simulink model "sampleModel2072_pp_difftest"  (R2021a)
settings: Solver=VariableStepAuto  StartTime=0.0  StopTime=10.0  RelTol=1e-3
undefined symbols (not defined in the file or in its folder): DiscIntNeverNeededParam, magnitude, Newton, Raphson
libraries: simulink x184, pid_lib x33
(part 4 of 5)

== system sampleModel2072_pp_difftest/cfblk49/cfblk12 ==
  cfblk1 : Inport
  cfblk3 : pid_lib/PID Controller  Controller=PID  Form=Parallel  TimeDomain=Discrete-time  UseExternalTs=off  SampleTime=1  IntegratorMethod=Forward Euler  FilterMethod=Forward Euler  ControllerParametersSource=internal  P=1  I=1  D=0  UseFilter=on  N=100  TunerSelectOption=Transfer Function Based (PID Tuner App)  InitialConditionSource=internal  InitialConditionForIntegrator=0  InitialConditionForFilter=0  DifferentiatorICPrevScaledInput=0  ExternalReset=none  TrackingMode=off  Kt=1  LimitOutput=off  SatLimitsSource=internal  UpperSaturationLimit=inf  LowerSaturationLimit=-inf  LinearizeAsGain=off  AntiWindupMode=none  Kb=1  POutMin=[]  POutMax=[]  IOutMin=[]  IOutMax=[]  DOutMin=[]  DOutMax=[]  NOutMin=[]  NOutMax=[]  SumOutMin=[]  SumOutMax=[]  SaturationOutMin=[]  SaturationOutMax=[]  PParamMin=[]  PParamMax=[]  IParamMin=[]  IParamMax=[]  DParamMin=[]  DParamMax=[]  NParamMin=[]  NParamMax=[]  KbParamMin=[]  KbParamMax=[]  KtParamMin=[]  KtParamMax=[]  KbOutMin=[]  KbOutMax=[]  KtOutMin=[]  KtOutMax=[]  IntegratorOutMin=[]  IntegratorOutMax=[]  FilterOutMin=[]  FilterOutMax=[]  SumI1OutMin=[]  SumI1OutMax=[]  SumI2OutMin=[]  SumI2OutMax=[]  SumI3OutMin=[]  SumI3OutMax=[]  SumI4OutMin=[]  SumI4OutMax=[]  SumDOutMin=[]  SumDOutMax=[]  DifferentiatorOutMin=[]  DifferentiatorOutMax=[]  FilterDiffOutCoefMin=[]  FilterDiffOutCoefMax=[]  ReciprocalOutMin=[]  ReciprocalOutMax=[]  SumDenOutMin=[]  SumDenOutMax=[]  SumNumOutMin=[]  SumNumOutMax=[]  DivideOutMin=[]  DivideOutMax=[]  UdiffTsProdOutMin=[]  UdiffTsProdOutMax=[]  NTsProdOutMin=[]  NTsProdOutMax=[]  UintegralTsProdOutMin=[]  UintegralTsProdOutMax=[]  UngainTsProdOutMin=[]  UngainTsProdOutMax=[]  IntegratorContinuousStateAttributes=''  IntegratorStateMustResolveToSignalObject=off  IntegratorRTWStateStorageClass=Auto  FilterContinuousStateAttributes=''  FilterStateMustResolveToSignalObject=off  FilterRTWStateStorageClass=Auto  ParallelPVariant=InternalParameters  IdealPVariant=Disabled  IVariant=InternalParameters  DVariant=InternalParameters  IntegratorVariant=Discrete  SatVariant=Disabled  AWVariant=Passthrough  PCopyVariant=Disabled  TRVariant=Disabled  FdbkBlocksVariant=Forward  IdealPFdbkVariant=Disabled  SatFdbkVariant=Disabled  DerivativeFilterVariant=ForwardEulerFilter  NVariant=InternalParameters  NCopyVariant=Disabled  FilterICVariant=InternalICsFilter  IntegratorICVariant=InternalICs  ExternalResetVariant=Disabled  TRSumVariant=Passthrough  SumFdbkVariant=Disabled  SumVariant=Sum_PID  TsampFilterVariant=InternalTs  TsampNgainVariant=Passthrough  TsampIntegralVariant=Passthrough  ExternalSaturationOutDataTypeStr=Inherit: Same as second input
  cfblk4 : simulink/Discrete/Transfer Fcn Lead or Lag  PoleZ=0.95  ZeroZ=0.75  ICPrevOutput=0.0  ICPrevInput=0.0  DoSatur=off
      settings: SourceProductBaseCode=SL
  cfblk5 : Abs
  cfblk6 : Math  Operator=mod  SaturateOnIntegerOverflow=on
  cfblk7 : Squeeze
  cfblk8 : Delay  SampleTime=1
  cfblk2 : Outport
  wires:
  cfblk6/1 -> cfblk3/1
  cfblk5/1 -> cfblk2/1
  cfblk3/1 -> cfblk7/1
  cfblk7/1 -> cfblk4/1, cfblk5/1
  cfblk1/1 -> cfblk6/2
  cfblk4/1 -> cfblk8/1
  cfblk8/1 -> cfblk6/1

== system sampleModel2072_pp_difftest/cfblk49/cfblk13 ==
  cfblk1 : Inport
  cfblk3 : DiscreteTransferFcn  SampleTime=1
  cfblk4 : simulink/Discrete/Difference  ICPrevInput=0.0  OutMin=[]  OutMax=[]  OutDataTypeStr=Inherit: Inherit via back propagation  OutDataType=fixdt(1, 16)  OutScaling=2^-10  DoSatur=off
  cfblk5 : Polyval  Coefs=[ +2.081618890e-019, -1.441693666e-014, +4.719686976e-010, -8.536869453e-006, +1.621573104e-001, -8.087801117e+001 ]
  cfblk6 : Product  Inputs=**
  cfblk7 : MinMax
  cfblk8 : Sin  TimeSource=Use external signal  SampleTime=0
  cfblk9 : Constant  Value=[-889653633.727904]  SampleTime=1
  cfblk2 : Outport
  wires:
  cfblk1/1 -> cfblk6/1
  cfblk9/1 -> cfblk3/1
  cfblk7/1 -> cfblk6/2
  cfblk6/1 -> cfblk2/1
  cfblk8/1 -> cfblk7/1
  cfblk3/1 -> cfblk5/1, cfblk4/1
  cfblk5/1 -> cfblk8/1

== system sampleModel2072_pp_difftest/cfblk49/cfblk14 ==
  cfblk1 : Inport
  cfblk10 : ComplexToRealImag
  cfblk11 : Polyval  Coefs=[ +2.081618890e-019, -1.441693666e-014, +4.719686976e-010, -8.536869453e-006, +1.621573104e-001, -8.087801117e+001 ]
  cfblk12 : Product
  cfblk13 : Reshape
  cfblk14 : Delay  SampleTime=1
  cfblk15 : Delay  SampleTime=1
  cfblk3 : DiscreteStateSpace
  cfblk4 : pid_lib/PID Controller (2DOF)  Controller=PID  Form=Parallel  TimeDomain=Discrete-time  UseExternalTs=off  SampleTime=1  IntegratorMethod=Forward Euler  FilterMethod=Forward Euler  ControllerParametersSource=internal  P=1  I=1  D=0  UseFilter=on  N=100  b=1  c=1  TunerSelectOption=Transfer Function Based (PID Tuner App)  InitialConditionSource=internal  InitialConditionForIntegrator=0  InitialConditionForFilter=0  DifferentiatorICPrevScaledInput=0  ExternalReset=none  TrackingMode=off  Kt=1  LimitOutput=off  SatLimitsSource=internal  UpperSaturationLimit=inf  LowerSaturationLimit=-inf  LinearizeAsGain=off  AntiWindupMode=none  Kb=1  POutMin=[]  POutMax=[]  IOutMin=[]  IOutMax=[]  DOutMin=[]  DOutMax=[]  NOutMin=[]  NOutMax=[]  bOutMin=[]  bOutMax=[]  cOutMin=[]  cOutMax=[]  SumOutMin=[]  SumOutMax=[]  SaturationOutMin=[]  SaturationOutMax=[]  PParamMin=[]  PParamMax=[]  IParamMin=[]  IParamMax=[]  DParamMin=[]  DParamMax=[]  NParamMin=[]  NParamMax=[]  bParamMin=[]  bParamMax=[]  cParamMin=[]  cParamMax=[]  KbParamMin=[]  KbParamMax=[]  KtParamMin=[]  KtParamMax=[]  KbOutMin=[]  KbOutMax=[]  KtOutMin=[]  KtOutMax=[]  IntegratorOutMin=[]  IntegratorOutMax=[]  FilterOutMin=[]  FilterOutMax=[]  SumI1OutMin=[]  SumI1OutMax=[]  SumI2OutMin=[]  SumI2OutMax=[]  SumI3OutMin=[]  SumI3OutMax=[]  SumI4OutMin=[]  SumI4OutMax=[]  SumDOutMin=[]  SumDOutMax=[]  Sum1OutMin=[]  Sum1OutMax=[]  Sum2OutMin=[]  Sum2OutMax=[]  Sum3OutMin=[]  Sum3OutMax=[]  DifferentiatorOutMin=[]  DifferentiatorOutMax=[]  FilterDiffOutCoefMin=[]  FilterDiffOutCoefMax=[]  ReciprocalOutMin=[]  ReciprocalOutMax=[]  SumDenOutMin=[]  SumDenOutMax=[]  SumNumOutMin=[]  SumNumOutMax=[]  DivideOutMin=[]  DivideOutMax=[]  UdiffTsProdOutMin=[]  UdiffTsProdOutMax=[]  NTsProdOutMin=[]  NTsProdOutMax=[]  UintegralTsProdOutMin=[]  UintegralTsProdOutMax=[]  UngainTsProdOutMin=[]  UngainTsProdOutMax=[]  IntegratorContinuousStateAttributes=''  IntegratorStateMustResolveToSignalObject=off  IntegratorRTWStateStorageClass=Auto  FilterContinuousStateAttributes=''  FilterStateMustResolveToSignalObject=off  FilterRTWStateStorageClass=Auto  ParallelPVariant=InternalParameters  IdealPVariant=Disabled  IVariant=InternalParameters  DVariant=InternalParameters  bVariant=InternalParameters  cVariant=InternalParameters  IntegratorVariant=Discrete  SatVariant=Disabled  AWVariant=Passthrough  PCopyVariant=Disabled  TRVariant=Disabled  FdbkBlocksVariant=Forward  IdealPFdbkVariant=Disabled  SatFdbkVariant=Disabled  DerivativeFilterVariant=ForwardEulerFilter  NVariant=InternalParameters  NCopyVariant=Disabled  FilterICVariant=InternalICsFilter  IntegratorICVariant=InternalICs  ExternalResetVariant=Disabled  TRSumVariant=Passthrough  SumFdbkVariant=Disabled  SumVariant=Sum_PID  TsampFilterVariant=InternalTs  TsampNgainVariant=Passthrough  TsampIntegralVariant=Passthrough  ExternalSaturationOutDataTypeStr=Inherit: Same as second input
      settings: SourceProductBaseCode=SL
  cfblk5 : simulink/Discrete/Transfer Fcn Real Zero  ZeroZ=0.75  ICPrevInput=0.0  DoSatur=off
      settings: SourceProductBaseCode=SL
  cfblk6 : Gain  Gain=[-781160074.490628]
  cfblk7 : Rounding
  cfblk8 : Abs
  cfblk9 : Sin  TimeSource=Use external signal  SampleTime=0
  cfblk2 : Outport
  wires:
  cfblk8/1 -> cfblk10/1
  cfblk5/1 -> cfblk13/1
  cfblk9/1 -> cfblk8/1
  cfblk4/1 -> cfblk2/1
  cfblk13/1 -> cfblk3/1, cfblk9/1
  cfblk6/1 -> cfblk4/1
  cfblk1/1 -> cfblk6/1
  cfblk11/1 -> cfblk7/1
  cfblk3/1 -> cfblk12/1
  cfblk12/1 -> cfblk11/1
  cfblk10/2 -> cfblk4/2
  cfblk7/1 -> cfblk14/1
  cfblk14/1 -> cfblk12/2
  cfblk10/1 -> cfblk15/1
  cfblk15/1 -> cfblk5/1

== system sampleModel2072_pp_difftest/cfblk49/cfblk15 ==
  cfblk1 : Inport
  cfblk11 : Inport  Port=2
  cfblk10 : Signum
  cfblk3 : UnitDelay  HasFrameUpgradeWarning=on
  cfblk4 : DiscreteFir  SampleTime=1
  cfblk5 : DiscreteZeroPole  Poles=[0 0.5]  Gain=1
  cfblk6 : Squeeze
  cfblk7 : Sqrt  SaturateOnIntegerOverflow=on
  cfblk8 : Squeeze
  cfblk9 : UnaryMinus
  cfblk2 : Outport
  wires:
  cfblk10/1 -> cfblk4/1
  cfblk3/1 -> cfblk2/1
  cfblk1/1 -> cfblk7/1
  cfblk8/1 -> cfblk5/1
  cfblk11/1 -> cfblk10/1
  cfblk5/1 -> cfblk9/1
  cfblk6/1 -> cfblk8/1
  cfblk7/1 -> cfblk6/1
  cfblk9/1 -> cfblk3/1

== system sampleModel2072_pp_difftest/cfblk49/cfblk16 ==
  cfblk1 : Inport
  cfblk10 : PermuteDimensions
  cfblk11 : Sum  Inputs=+
  cfblk12 : UnaryMinus
  cfblk13 : Sum  Inputs=+-
  cfblk14 : simulink/Math Operations/MinMax Running Resettable  Function=min  vinit=0.0
  cfblk15 : Reshape
  cfblk16 : Gain  Gain=[569641442.410553]
  cfblk17 : Delay  SampleTime=1
  cfblk18 : Delay  SampleTime=1
  cfblk3 : pid_lib/PID Controller (2DOF)  Controller=PID  Form=Parallel  TimeDomain=Discrete-time  UseExternalTs=off  SampleTime=1  IntegratorMethod=Forward Euler  FilterMethod=Forward Euler  ControllerParametersSource=internal  P=1  I=1  D=0  UseFilter=on  N=100  b=1  c=1  TunerSelectOption=Transfer Function Based (PID Tuner App)  InitialConditionSource=internal  InitialConditionForIntegrator=0  InitialConditionForFilter=0  DifferentiatorICPrevScaledInput=0  ExternalReset=none  TrackingMode=off  Kt=1  LimitOutput=off  SatLimitsSource=internal  UpperSaturationLimit=inf  LowerSaturationLimit=-inf  LinearizeAsGain=off  AntiWindupMode=none  Kb=1  POutMin=[]  POutMax=[]  IOutMin=[]  IOutMax=[]  DOutMin=[]  DOutMax=[]  NOutMin=[]  NOutMax=[]  bOutMin=[]  bOutMax=[]  cOutMin=[]  cOutMax=[]  SumOutMin=[]  SumOutMax=[]  SaturationOutMin=[]  SaturationOutMax=[]  PParamMin=[]  PParamMax=[]  IParamMin=[]  IParamMax=[]  DParamMin=[]  DParamMax=[]  NParamMin=[]  NParamMax=[]  bParamMin=[]  bParamMax=[]  cParamMin=[]  cParamMax=[]  KbParamMin=[]  KbParamMax=[]  KtParamMin=[]  KtParamMax=[]  KbOutMin=[]  KbOutMax=[]  KtOutMin=[]  KtOutMax=[]  IntegratorOutMin=[]  IntegratorOutMax=[]  FilterOutMin=[]  FilterOutMax=[]  SumI1OutMin=[]  SumI1OutMax=[]  SumI2OutMin=[]  SumI2OutMax=[]  SumI3OutMin=[]  SumI3OutMax=[]  SumI4OutMin=[]  SumI4OutMax=[]  SumDOutMin=[]  SumDOutMax=[]  Sum1OutMin=[]  Sum1OutMax=[]  Sum2OutMin=[]  Sum2OutMax=[]  Sum3OutMin=[]  Sum3OutMax=[]  DifferentiatorOutMin=[]  DifferentiatorOutMax=[]  FilterDiffOutCoefMin=[]  FilterDiffOutCoefMax=[]  ReciprocalOutMin=[]  ReciprocalOutMax=[]  SumDenOutMin=[]  SumDenOutMax=[]  SumNumOutMin=[]  SumNumOutMax=[]  DivideOutMin=[]  DivideOutMax=[]  UdiffTsProdOutMin=[]  UdiffTsProdOutMax=[]  NTsProdOutMin=[]  NTsProdOutMax=[]  UintegralTsProdOutMin=[]  UintegralTsProdOutMax=[]  UngainTsProdOutMin=[]  UngainTsProdOutMax=[]  IntegratorContinuousStateAttributes=''  IntegratorStateMustResolveToSignalObject=off  IntegratorRTWStateStorageClass=Auto  FilterContinuousStateAttributes=''  FilterStateMustResolveToSignalObject=off  FilterRTWStateStorageClass=Auto  ParallelPVariant=InternalParameters  IdealPVariant=Disabled  IVariant=InternalParameters  DVariant=InternalParameters  bVariant=InternalParameters  cVariant=InternalParameters  IntegratorVariant=Discrete  SatVariant=Disabled  AWVariant=Passthrough  PCopyVariant=Disabled  TRVariant=Disabled  FdbkBlocksVariant=Forward  IdealPFdbkVariant=Disabled  SatFdbkVariant=Disabled  DerivativeFilterVariant=ForwardEulerFilter  NVariant=InternalParameters  NCopyVariant=Disabled  FilterICVariant=InternalICsFilter  IntegratorICVariant=InternalICs  ExternalResetVariant=Disabled  TRSumVariant=Passthrough  SumFdbkVariant=Disabled  SumVariant=Sum_PID  TsampFilterVariant=InternalTs  TsampNgainVariant=Passthrough  TsampIntegralVariant=Passthrough  ExternalSaturationOutDataTypeStr=Inherit: Same as second input
      settings: SourceProductBaseCode=SL
  cfblk4 : Delay  ShowEnablePort=on  SampleTime=1
      settings: InputPortMap=u0,e6
  cfblk5 : DiscreteIntegrator  ICPrevOutput=DiscIntNeverNeededParam  ICPrevScaledInput=DiscIntNeverNeededParam
  cfblk6 : UnitDelay  HasFrameUpgradeWarning=on
  cfblk7 : Delay  ShowEnablePort=on  SampleTime=1
      settings: InputPortMap=u0,e6
  cfblk8 : Reshape
  cfblk9 : simulink/Math Operations/Slider Gain  gain=1  low=0  high=2
  cfblk2 : Outport
  wires:
  cfblk4/1 -> cfblk5/1
  cfblk14/1 -> cfblk3/1
  cfblk1/1 -> cfblk16/1, cfblk14/2
  cfblk9/1 -> cfblk11/1, cfblk8/1
  cfblk5/1 -> cfblk12/1
  cfblk8/1 -> cfblk7/1, cfblk7/2
  cfblk12/1 -> cfblk6/1
  cfblk16/1 -> cfblk3/2
  cfblk11/1 -> cfblk4/1, cfblk15/1
  cfblk13/1 -> cfblk2/1
  cfblk10/1 -> cfblk13/1
  cfblk7/1 -> cfblk14/1
  cfblk3/1 -> cfblk10/1
  cfblk6/1 -> cfblk13/2, cfblk17/1
  cfblk17/1 -> cfblk4/2
  cfblk15/1 -> cfblk18/1
  cfblk18/1 -> cfblk9/1

== system sampleModel2072_pp_difftest/cfblk49/cfblk18 ==
  cfblk1 : Inport
  cfblk15 : Inport  Port=2
  Action Port : ActionPort  ActionPortLabel=if(u1 >= 0)
  cfblk10 : UnaryMinus
  cfblk11 : Signum
  cfblk12 : Bias  Bias=[-787448639.823052]
  cfblk13 : DotProduct  InputSameDT=on  OutDataTypeStr=Inherit: Inherit via internal rule
  cfblk14 : Constant  Value=[137570796.865907]  SampleTime=1
  cfblk16 : Delay
  cfblk17 : Delay
  cfblk3 : simulink/Discrete/Tapped Delay  vinit=0.0  samptime=-1  NumDelays=1  DelayOrder=Oldest  includeCurrent=off
  cfblk4 : DiscreteFir
  cfblk5 : simulink/Discrete/Transfer Fcn Lead or Lag  PoleZ=0.95  ZeroZ=0.75  ICPrevOutput=0.0  ICPrevInput=0.0  DoSatur=off
      settings: SourceProductBaseCode=SL
  cfblk6 : Product  Inputs=**
  cfblk7 : Polyval  Coefs=[ +2.081618890e-019, -1.441693666e-014, +4.719686976e-010, -8.536869453e-006, +1.621573104e-001, -8.087801117e+001 ]
  cfblk8 : simulink/Math Operations/MinMax Running Resettable  Function=min  vinit=0.0
  cfblk9 : Squeeze
  cfblk2 : Outport
  wires:
  cfblk8/1 -> cfblk3/1
  cfblk13/1 -> cfblk7/1
  cfblk6/1 -> cfblk4/1
  cfblk10/1 -> cfblk2/1, cfblk16/1
  cfblk7/1 -> cfblk12/1
  cfblk4/1 -> cfblk10/1
  cfblk1/1 -> cfblk6/1
  cfblk15/1 -> cfblk11/1
  cfblk3/1 -> cfblk5/1
  cfblk5/1 -> cfblk9/1
  cfblk9/1 -> cfblk13/1
  cfblk11/1 -> cfblk8/1
  cfblk14/1 -> cfblk8/2
  cfblk16/1 -> cfblk6/2
  cfblk12/1 -> cfblk17/1
  cfblk17/1 -> cfblk13/2

== system sampleModel2072_pp_difftest/cfblk49/cfblk19 ==
  cfblk1 : Inport
  Action Port : ActionPort  ActionPortLabel=else
  cfblk10 : Sqrt  SaturateOnIntegerOverflow=on
  cfblk11 : Polyval  Coefs=[ +2.081618890e-019, -1.441693666e-014, +4.719686976e-010, -8.536869453e-006, +1.621573104e-001, -8.087801117e+001 ]
  cfblk12 : Product
  cfblk13 : Abs
  cfblk14 : Delay
  cfblk15 : Delay
  cfblk3 : DiscreteZeroPole  Poles=[0 0.5]  Gain=1  SampleTime=-1
  cfblk4 : Delay
  cfblk5 : DiscreteStateSpace  SampleTime=-1
  cfblk6 : Sum  Inputs=+-
  cfblk7 : Sqrt  Operator=rSqrt  AlgorithmType=Newton-Raphson  SaturateOnIntegerOverflow=on
  cfblk8 : Polyval  Coefs=[ +2.081618890e-019, -1.441693666e-014, +4.719686976e-010, -8.536869453e-006, +1.621573104e-001, -8.087801117e+001 ]
  cfblk9 : Sum  Inputs=+
  cfblk2 : Outport
  wires:
  cfblk5/1 -> cfblk9/1, cfblk4/1
  cfblk13/1 -> cfblk11/1
  cfblk12/1 -> cfblk13/1
  cfblk1/1 -> cfblk7/1
  cfblk8/1 -> cfblk2/1
  cfblk4/1 -> cfblk8/1
  cfblk7/1 -> cfblk10/1
  cfblk10/1 -> cfblk6/1, cfblk6/2
  cfblk6/1 -> cfblk12/2
  cfblk11/1 -> cfblk3/1
  cfblk3/1 -> cfblk14/1
  cfblk14/1 -> cfblk12/1
  cfblk9/1 -> cfblk15/1
  cfblk15/1 -> cfblk5/1

== system sampleModel2072_pp_difftest/cfblk51/cfblk6 ==
  cfblk1 : Inport
  cfblk10 : Sqrt  SaturateOnIntegerOverflow=on
  cfblk11 : Sqrt  SaturateOnIntegerOverflow=on
  cfblk12 : Assignment  DiagnosticForDimensions=Warning  IndexOptions=Index vector (dialog)  Indices=1  OutputSizes=1
  cfblk13 : Sqrt  SaturateOnIntegerOverflow=on
  cfblk14 : Product  Inputs=*
  cfblk15 : Delay  SampleTime=1
  cfblk16 : Delay  SampleTime=1
  cfblk17 : Delay  SampleTime=1
  cfblk3 : DiscreteStateSpace
  cfblk4 : DiscreteFir  SampleTime=1
  cfblk5 : pid_lib/PID Controller (2DOF)  Controller=PID  Form=Parallel  TimeDomain=Discrete-time  UseExternalTs=off  SampleTime=1  IntegratorMethod=Forward Euler  FilterMethod=Forward Euler  ControllerParametersSource=internal  P=1  I=1  D=0  UseFilter=on  N=100  b=1  c=1  TunerSelectOption=Transfer Function Based (PID Tuner App)  InitialConditionSource=internal  InitialConditionForIntegrator=0  InitialConditionForFilter=0  DifferentiatorICPrevScaledInput=0  ExternalReset=none  TrackingMode=off  Kt=1  LimitOutput=off  SatLimitsSource=internal  UpperSaturationLimit=inf  LowerSaturationLimit=-inf  LinearizeAsGain=off  AntiWindupMode=none  Kb=1  POutMin=[]  POutMax=[]  IOutMin=[]  IOutMax=[]  DOutMin=[]  DOutMax=[]  NOutMin=[]  NOutMax=[]  bOutMin=[]  bOutMax=[]  cOutMin=[]  cOutMax=[]  SumOutMin=[]  SumOutMax=[]  SaturationOutMin=[]  SaturationOutMax=[]  PParamMin=[]  PParamMax=[]  IParamMin=[]  IParamMax=[]  DParamMin=[]  DParamMax=[]  NParamMin=[]  NParamMax=[]  bParamMin=[]  bParamMax=[]  cParamMin=[]  cParamMax=[]  KbParamMin=[]  KbParamMax=[]  KtParamMin=[]  KtParamMax=[]  KbOutMin=[]  KbOutMax=[]  KtOutMin=[]  KtOutMax=[]  IntegratorOutMin=[]  IntegratorOutMax=[]  FilterOutMin=[]  FilterOutMax=[]  SumI1OutMin=[]  SumI1OutMax=[]  SumI2OutMin=[]  SumI2OutMax=[]  SumI3OutMin=[]  SumI3OutMax=[]  SumI4OutMin=[]  SumI4OutMax=[]  SumDOutMin=[]  SumDOutMax=[]  Sum1OutMin=[]  Sum1OutMax=[]  Sum2OutMin=[]  Sum2OutMax=[]  Sum3OutMin=[]  Sum3OutMax=[]  DifferentiatorOutMin=[]  DifferentiatorOutMax=[]  FilterDiffOutCoefMin=[]  FilterDiffOutCoefMax=[]  ReciprocalOutMin=[]  ReciprocalOutMax=[]  SumDenOutMin=[]  SumDenOutMax=[]  SumNumOutMin=[]  SumNumOutMax=[]  DivideOutMin=[]  DivideOutMax=[]  UdiffTsProdOutMin=[]  UdiffTsProdOutMax=[]  NTsProdOutMin=[]  NTsProdOutMax=[]  UintegralTsProdOutMin=[]  UintegralTsProdOutMax=[]  UngainTsProdOutMin=[]  UngainTsProdOutMax=[]  IntegratorContinuousStateAttributes=''  IntegratorStateMustResolveToSignalObject=off  IntegratorRTWStateStorageClass=Auto  FilterContinuousStateAttributes=''  FilterStateMustResolveToSignalObject=off  FilterRTWStateStorageClass=Auto  ParallelPVariant=InternalParameters  IdealPVariant=Disabled  IVariant=InternalParameters  DVariant=InternalParameters  bVariant=InternalParameters  cVariant=InternalParameters  IntegratorVariant=Discrete  SatVariant=Disabled  AWVariant=Passthrough  PCopyVariant=Disabled  TRVariant=Disabled  FdbkBlocksVariant=Forward  IdealPFdbkVariant=Disabled  SatFdbkVariant=Disabled  DerivativeFilterVariant=ForwardEulerFilter  NVariant=InternalParameters  NCopyVariant=Disabled  FilterICVariant=InternalICsFilter  IntegratorICVariant=InternalICs  ExternalResetVariant=Disabled  TRSumVariant=Passthrough  SumFdbkVariant=Disabled  SumVariant=Sum_PID  TsampFilterVariant=InternalTs  TsampNgainVariant=Passthrough  TsampIntegralVariant=Passthrough  ExternalSaturationOutDataTypeStr=Inherit: Same as second input
      settings: SourceProductBaseCode=SL
  cfblk6 : simulink/Discrete/Transfer Fcn First Order  PoleZ=0.95  ICPrevOutput=0.0  DoSatur=off
  cfblk7 : Product  Inputs=**
  cfblk8 : PermuteDimensions
  cfblk9 : Bias  Bias=[-648568228.992843]
  cfblk2 : Outport
  wires:
  cfblk7/1 -> cfblk11/1
  cfblk6/1 -> cfblk4/1
  cfblk13/1 -> cfblk6/1, cfblk17/1
  cfblk8/1 -> cfblk13/1
  cfblk9/1 -> cfblk5/1
  cfblk14/1 -> cfblk7/1
  cfblk12/1 -> cfblk3/1
  cfblk3/1 -> cfblk9/1
  cfblk4/1 -> cfblk2/1, cfblk5/2
  cfblk1/1 -> cfblk10/1, cfblk12/2
  cfblk10/1 -> cfblk14/1
  cfblk11/1 -> cfblk15/1
  cfblk15/1 -> cfblk7/2
  cfblk5/1 -> cfblk16/1
  cfblk16/1 -> cfblk12/1
  cfblk17/1 -> cfblk8/1

== system sampleModel2072_pp_difftest/cfblk51/cfblk7 ==
  cfblk1 : Inport
  cfblk10 : Delay  SampleTime=1
  cfblk3 : DiscreteFilter  SampleTime=1
  cfblk4 : Sum  Inputs=+-
  cfblk5 : Sqrt  Operator=rSqrt  AlgorithmType=Newton-Raphson  SaturateOnIntegerOverflow=on
  cfblk6 : Sum  Inputs=+-
  cfblk7 : ComplexToMagnitudeAngle
  cfblk8 : DotProduct  InputSameDT=on  OutDataTypeStr=Inherit: Inherit via internal rule
  cfblk9 : Delay  SampleTime=1
  cfblk2 : Outport
  wires:
  cfblk4/1 -> cfblk5/1
  cfblk7/1 -> cfblk6/1
  cfblk3/1 -> cfblk4/1
  cfblk8/1 -> cfblk2/1
  cfblk1/1 -> cfblk6/2, cfblk8/2
  cfblk6/1 -> cfblk8/1
  cfblk5/1 -> cfblk7/1, cfblk10/1
  cfblk7/2 -> cfblk9/1
  cfblk9/1 -> cfblk3/1
  cfblk10/1 -> cfblk4/2

== system sampleModel2072_pp_difftest/cfblk51/cfblk8 ==
  cfblk1 : Inport
  cfblk10 : Reshape
  cfblk11 : Delay  SampleTime=1
  cfblk3 : DiscreteStateSpace
  cfblk4 : Signum
  cfblk5 : Squeeze
  cfblk6 : Sum  Inputs=+
  cfblk7 : Math  Operator=hypot  SaturateOnIntegerOverflow=on
  cfblk8 : Reshape
  cfblk9 : ComplexToMagnitudeAngle
  cfblk2 : Outport
  wires:
  cfblk1/1 -> cfblk9/1
  cfblk5/1 -> cfblk8/1
  cfblk6/1 -> cfblk3/1
  cfblk4/1 -> cfblk5/1
  cfblk9/1 -> cfblk2/1
  cfblk8/1 -> cfblk10/1
  cfblk10/1 -> cfblk7/1
  cfblk9/2 -> cfblk4/1
  cfblk7/1 -> cfblk6/1
  cfblk3/1 -> cfblk11/1
  cfblk11/1 -> cfblk7/2

== system sampleModel2072_pp_difftest/cfblk51/cfblk9 ==
  cfblk1 : Inport
  cfblk10 : Sum  Inputs=+
  cfblk11 : ComplexToMagnitudeAngle
  cfblk12 : Sum  Inputs=|++
  cfblk13 : Sin  TimeSource=Use external signal  SampleTime=0
  cfblk14 : Polyval  Coefs=[ +2.081618890e-019, -1.441693666e-014, +4.719686976e-010, -8.536869453e-006, +1.621573104e-001, -8.087801117e+001 ]
  cfblk15 : Delay  SampleTime=1
  cfblk16 : Delay  SampleTime=1
  cfblk17 : Delay  SampleTime=1
  cfblk3 : simulink/Discrete/Transfer Fcn Real Zero  ZeroZ=0.75  ICPrevInput=0.0  DoSatur=off
      settings: SourceProductBaseCode=SL
  cfblk4 : DiscreteTransferFcn  SampleTime=1
  cfblk5 : Sum  Inputs=|++
  cfblk6 : Sqrt  SaturateOnIntegerOverflow=on
  cfblk7 : Gain  Gain=[-400651424.517139]
  cfblk8 : Product  Inputs=*
  cfblk9 : Sum  Inputs=+-
  cfblk2 : Outport
  wires:
  cfblk4/1 -> cfblk13/1
  cfblk7/1 -> cfblk9/1
  cfblk14/1 -> cfblk3/1
  cfblk5/1 -> cfblk14/1
  cfblk10/1 -> cfblk9/2
  cfblk6/1 -> cfblk11/1
  cfblk11/1 -> cfblk8/1
  cfblk11/2 -> cfblk7/1, cfblk2/1, cfblk17/1
  cfblk13/1 -> cfblk10/1
  cfblk8/1 -> cfblk12/1
  cfblk12/1 -> cfblk5/2
  cfblk1/1 -> cfblk12/2
  cfblk3/1 -> cfblk15/1
  cfblk15/1 -> cfblk5/1
  cfblk9/1 -> cfblk16/1
  cfblk16/1 -> cfblk4/1
  cfblk17/1 -> cfblk6/1

== system sampleModel2072_pp_difftest/cfblk52/cfblk13 ==
  cfblk1 : Inport
  cfblk10 : Trigonometry
  cfblk11 : simulink/Math Operations/Slider Gain  gain=1  low=0  high=2
  cfblk12 : Trigonometry
  cfblk13 : Math  Operator=10^u  SaturateOnIntegerOverflow=on
  cfblk14 : Delay  SampleTime=1
  cfblk3 : simulink/Discrete/Difference  ICPrevInput=0.0  OutMin=[]  OutMax=[]  OutDataTypeStr=Inherit: Inherit via back propagation  OutDataType=fixdt(1, 16)  OutScaling=2^-10  DoSatur=off
  cfblk4 : simulink/Discrete/Tapped Delay  vinit=0.0  samptime=-1  NumDelays=1  DelayOrder=Oldest  includeCurrent=off
  cfblk5 : pid_lib/PID Controller (2DOF)  Controller=PID  Form=Parallel  TimeDomain=Discrete-time  UseExternalTs=off  SampleTime=1  IntegratorMethod=Forward Euler  FilterMethod=Forward Euler  ControllerParametersSource=internal  P=1  I=1  D=0  UseFilter=on  N=100  b=1  c=1  TunerSelectOption=Transfer Function Based (PID Tuner App)  InitialConditionSource=internal  InitialConditionForIntegrator=0  InitialConditionForFilter=0  DifferentiatorICPrevScaledInput=0  ExternalReset=none  TrackingMode=off  Kt=1  LimitOutput=off  SatLimitsSource=internal  UpperSaturationLimit=inf  LowerSaturationLimit=-inf  LinearizeAsGain=off  AntiWindupMode=none  Kb=1  POutMin=[]  POutMax=[]  IOutMin=[]  IOutMax=[]  DOutMin=[]  DOutMax=[]  NOutMin=[]  NOutMax=[]  bOutMin=[]  bOutMax=[]  cOutMin=[]  cOutMax=[]  SumOutMin=[]  SumOutMax=[]  SaturationOutMin=[]  SaturationOutMax=[]  PParamMin=[]  PParamMax=[]  IParamMin=[]  IParamMax=[]  DParamMin=[]  DParamMax=[]  NParamMin=[]  NParamMax=[]  bParamMin=[]  bParamMax=[]  cParamMin=[]  cParamMax=[]  KbParamMin=[]  KbParamMax=[]  KtParamMin=[]  KtParamMax=[]  KbOutMin=[]  KbOutMax=[]  KtOutMin=[]  KtOutMax=[]  IntegratorOutMin=[]  IntegratorOutMax=[]  FilterOutMin=[]  FilterOutMax=[]  SumI1OutMin=[]  SumI1OutMax=[]  SumI2OutMin=[]  SumI2OutMax=[]  SumI3OutMin=[]  SumI3OutMax=[]  SumI4OutMin=[]  SumI4OutMax=[]  SumDOutMin=[]  SumDOutMax=[]  Sum1OutMin=[]  Sum1OutMax=[]  Sum2OutMin=[]  Sum2OutMax=[]  Sum3OutMin=[]  Sum3OutMax=[]  DifferentiatorOutMin=[]  DifferentiatorOutMax=[]  FilterDiffOutCoefMin=[]  FilterDiffOutCoefMax=[]  ReciprocalOutMin=[]  ReciprocalOutMax=[]  SumDenOutMin=[]  SumDenOutMax=[]  SumNumOutMin=[]  SumNumOutMax=[]  DivideOutMin=[]  DivideOutMax=[]  UdiffTsProdOutMin=[]  UdiffTsProdOutMax=[]  NTsProdOutMin=[]  NTsProdOutMax=[]  UintegralTsProdOutMin=[]  UintegralTsProdOutMax=[]  UngainTsProdOutMin=[]  UngainTsProdOutMax=[]  IntegratorContinuousStateAttributes=''  IntegratorStateMustResolveToSignalObject=off  IntegratorRTWStateStorageClass=Auto  FilterContinuousStateAttributes=''  FilterStateMustResolveToSignalObject=off  FilterRTWStateStorageClass=Auto  ParallelPVariant=InternalParameters  IdealPVariant=Disabled  IVariant=InternalParameters  DVariant=InternalParameters  bVariant=InternalParameters  cVariant=InternalParameters  IntegratorVariant=Discrete  SatVariant=Disabled  AWVariant=Passthrough  PCopyVariant=Disabled  TRVariant=Disabled  FdbkBlocksVariant=Forward  IdealPFdbkVariant=Disabled  SatFdbkVariant=Disabled  DerivativeFilterVariant=ForwardEulerFilter  NVariant=InternalParameters  NCopyVariant=Disabled  FilterICVariant=InternalICsFilter  IntegratorICVariant=InternalICs  ExternalResetVariant=Disabled  TRSumVariant=Passthrough  SumFdbkVariant=Disabled  SumVariant=Sum_PID  TsampFilterVariant=InternalTs  TsampNgainVariant=Passthrough  TsampIntegralVariant=Passthrough  ExternalSaturationOutDataTypeStr=Inherit: Same as second input
      settings: SourceProductBaseCode=SL
  cfblk6 : Sin  TimeSource=Use external signal  SampleTime=0
  cfblk7 : ComplexToRealImag
  cfblk8 : Sqrt  SaturateOnIntegerOverflow=on
  cfblk9 : ComplexToRealImag
  cfblk2 : Outport
  wires:
  cfblk1/1 -> cfblk4/1
  cfblk5/1 -> cfblk7/1
  cfblk10/1 -> cfblk12/1
  cfblk4/1 -> cfblk9/1
  cfblk13/1 -> cfblk6/1
  cfblk6/1 -> cfblk11/1
  cfblk11/1 -> cfblk8/1
  cfblk8/1 -> cfblk2/1
  cfblk7/1 -> cfblk13/1
  cfblk12/1 -> cfblk3/1
  cfblk9/1 -> cfblk5/2
  cfblk7/2 -> cfblk10/1
  cfblk3/1 -> cfblk14/1
  cfblk14/1 -> cfblk5/1

== system sampleModel2072_pp_difftest/cfblk52/cfblk14 ==
  cfblk1 : Inport
  cfblk3 : Product
  cfblk4 : Rounding
  cfblk5 : Sum  Inputs=+-
  cfblk6 : simulink/Math Operations/Slider Gain  gain=1  low=0  high=2
  cfblk7 : Product  Inputs=*
  cfblk8 : Delay  SampleTime=1
  cfblk9 : Delay  SampleTime=1
  cfblk2 : Outport
  wires:
  cfblk7/1 -> cfblk6/1
  cfblk1/1 -> cfblk2/1, cfblk5/2
  cfblk5/1 -> cfblk3/1
  cfblk4/1 -> cfblk7/1, cfblk3/2
  cfblk3/1 -> cfblk8/1
  cfblk8/1 -> cfblk5/1
  cfblk6/1 -> cfblk9/1
  cfblk9/1 -> cfblk4/1

== system sampleModel2072_pp_difftest/cfblk52/cfblk15 ==
  cfblk1 : Inport
  cfblk10 : Constant  Value=[-219498579.036000]  SampleTime=1
  cfblk3 : simulink/Discrete/Transfer Fcn First Order  PoleZ=0.95  ICPrevOutput=0.0  DoSatur=off
  cfblk4 : Polyval  Coefs=[ +2.081618890e-019, -1.441693666e-014, +4.719686976e-010, -8.536869453e-006, +1.621573104e-001, -8.087801117e+001 ]
  cfblk5 : Reshape
  cfblk6 : Polyval  Coefs=[ +2.081618890e-019, -1.441693666e-014, +4.719686976e-010, -8.536869453e-006, +1.621573104e-001, -8.087801117e+001 ]
  cfblk7 : Sin  TimeSource=Use external signal  SampleTime=0
  cfblk8 : Sqrt  Operator=rSqrt  AlgorithmType=Newton-Raphson  SaturateOnIntegerOverflow=on
  cfblk9 : Gain  Gain=[907253447.135554]
  cfblk2 : Outport
  wires:
  cfblk6/1 -> cfblk2/1
  cfblk3/1 -> cfblk5/1
  cfblk10/1 -> cfblk7/1
  cfblk5/1 -> cfblk8/1
  cfblk4/1 -> cfblk9/1
  cfblk8/1 -> cfblk6/1
  cfblk7/1 -> cfblk4/1
  cfblk1/1 -> cfblk3/1

== system sampleModel2072_pp_difftest/cfblk53/cfblk10 ==
  cfblk1 : Inport
  cfblk13 : Inport  Port=2
  cfblk10 : Polyval  Coefs=[ +2.081618890e-019, -1.441693666e-014, +4.719686976e-010, -8.536869453e-006, +1.621573104e-001, -8.087801117e+001 ]
  cfblk11 : Product  Inputs=**
  cfblk12 : Sum  Inputs=+
  cfblk14 : Delay  SampleTime=1
  cfblk3 : DiscreteFilter  SampleTime=1
  cfblk4 : Sum  Inputs=+-
  cfblk5 : DotProduct  InputSameDT=on  OutDataTypeStr=Inherit: Inherit via internal rule
  cfblk6 : Product
  cfblk7 : Product  Inputs=*
  cfblk8 : Squeeze
  cfblk9 : Product  Inputs=*
  cfblk2 : Outport
  wires:
  cfblk9/1 -> cfblk7/1
  cfblk11/1 -> cfblk4/2
  cfblk13/1 -> cfblk10/1
  cfblk6/1 -> cfblk11/1
  cfblk10/1 -> cfblk9/1, cfblk6/2
  cfblk1/1 -> cfblk6/1
  cfblk4/1 -> cfblk8/1
  cfblk3/1 -> cfblk12/1
  cfblk7/1 -> cfblk5/1, cfblk3/1
  cfblk12/1 -> cfblk5/2, cfblk11/2
  cfblk5/1 -> cfblk2/1
  cfblk8/1 -> cfblk14/1
  cfblk14/1 -> cfblk4/1

== system sampleModel2072_pp_difftest/cfblk53/cfblk11 ==
  cfblk1 : Inport
  cfblk10 : MinMax  Function=max  Inputs=3
  cfblk11 : Signum
  cfblk12 : Gain  Gain=[481303857.511621]
  cfblk13 : Sum  Inputs=|++
  cfblk14 : Polyval  Coefs=[ +2.081618890e-019, -1.441693666e-014, +4.719686976e-010, -8.536869453e-006, +1.621573104e-001, -8.087801117e+001 ]
  cfblk15 : Abs
  cfblk{16..19} (4 alike) : Delay  SampleTime=1
  cfblk3 : Sqrt  Operator=rSqrt  AlgorithmType=Newton-Raphson  SaturateOnIntegerOverflow=on
  cfblk4 : Product
  cfblk5 : simulink/Math Operations/Slider Gain  gain=1  low=0  high=2
  cfblk6 : Bias  Bias=[-169922760.268926]
  cfblk7 : Signum
  cfblk8 : MinMax  Inputs=3
  cfblk9 : Signum
  cfblk2 : Outport
  wires:
  cfblk8/1 -> cfblk2/1, cfblk13/2, cfblk19/1
  cfblk10/1 -> cfblk15/1, cfblk8/3
  cfblk5/1 -> cfblk6/1
  cfblk7/1 -> cfblk10/1
  cfblk3/1 -> cfblk9/1
  cfblk12/1 -> cfblk5/1
  cfblk6/1 -> cfblk11/1
  cfblk13/1 -> cfblk14/1
  cfblk1/1 -> cfblk12/1
  cfblk4/1 -> cfblk7/1, cfblk10/3
  cfblk11/1 -> cfblk4/1
  cfblk14/1 -> cfblk3/1, cfblk18/1
  cfblk15/1 -> cfblk8/2, cfblk16/1
  cfblk16/1 -> cfblk10/2
  cfblk9/1 -> cfblk17/1
  cfblk17/1 -> cfblk8/1
  cfblk18/1 -> cfblk13/1
  cfblk19/1 -> cfblk4/2

== system sampleModel2072_pp_difftest/cfblk53/cfblk8 ==
  cfblk1 : Inport
  cfblk3 : DiscreteFir  SampleTime=1
  cfblk4 : Sum  Inputs=+-
  cfblk5 : ComplexToRealImag
  cfblk6 : ComplexToMagnitudeAngle
  cfblk7 : Polyval  Coefs=[ +2.081618890e-019, -1.441693666e-014, +4.719686976e-010, -8.536869453e-006, +1.621573104e-001, -8.087801117e+001 ]
  cfblk8 : Delay  SampleTime=1
  cfblk2 : Outport
  wires:
  cfblk1/1 -> cfblk2/1
  cfblk6/1 -> cfblk7/1
  cfblk5/1 -> cfblk4/1
  cfblk3/1 -> cfblk5/1
  cfblk6/2 -> cfblk4/2
  cfblk5/2 -> cfblk6/1
  cfblk7/1 -> cfblk8/1
  cfblk8/1 -> cfblk3/1

== system sampleModel2072_pp_difftest/cfblk53/cfblk9 ==
  cfblk1 : Inport
  cfblk10 : Polyval  Coefs=[ +2.081618890e-019, -1.441693666e-014, +4.719686976e-010, -8.536869453e-006, +1.621573104e-001, -8.087801117e+001 ]
  cfblk11 : Sin  TimeSource=Use external signal  SampleTime=0
  cfblk12 : Reshape
  cfblk13 : UnaryMinus
  cfblk14 : Sum  Inputs=+
  cfblk15 : PermuteDimensions
  cfblk16 : PermuteDimensions
  cfblk{3,17..19} (4 alike) : Delay  SampleTime=1
  cfblk4 : DiscreteFir  SampleTime=1
  cfblk5 : UnitDelay  HasFrameUpgradeWarning=on
  cfblk6 : Sum  Inputs=--
  cfblk7 : Sqrt  SaturateOnIntegerOverflow=on
  cfblk8 : ComplexToMagnitudeAngle
  cfblk9 : ComplexToMagnitudeAngle
  cfblk2 : Outport
  wires:
  cfblk15/1 -> cfblk9/1
  cfblk8/1 -> cfblk13/1
  cfblk6/1 -> cfblk15/1
  cfblk9/2 -> cfblk8/1
  cfblk7/1 -> cfblk14/1
  cfblk16/1 -> cfblk4/1
  cfblk14/1 -> cfblk12/1
  cfblk1/1 -> cfblk7/1
  cfblk4/1 -> cfblk11/1
  cfblk12/1 -> cfblk3/1
  cfblk5/1 -> cfblk10/1
  cfblk3/1 -> cfblk16/1
  cfblk11/1 -> cfblk2/1
  cfblk10/1 -> cfblk17/1
  cfblk17/1 -> cfblk5/1
  cfblk9/1 -> cfblk18/1
  cfblk18/1 -> cfblk6/1
  cfblk13/1 -> cfblk19/1
  cfblk19/1 -> cfblk6/2

== system sampleModel2072_pp_difftest/cfblk54/cfblk10 ==
  cfblk1 : Inport
  cfblk10 : ComplexToMagnitudeAngle
  cfblk11 : Reshape
  cfblk12 : Rounding
  cfblk13 : ComplexToRealImag
  cfblk14 : Constant  Value=[54363241.946083]  SampleTime=1
  cfblk15 : Delay  SampleTime=1
  cfblk3 : DiscreteFir  SampleTime=1
  cfblk4 : simulink/Discrete/Transfer Fcn First Order  PoleZ=0.95  ICPrevOutput=0.0  DoSatur=off
  cfblk5 : simulink/Discrete/Transfer Fcn Real Zero  ZeroZ=0.75  ICPrevInput=0.0  DoSatur=off
      settings: SourceProductBaseCode=SL
  cfblk6 : MinMax  Inputs=2
  cfblk7 : ComplexToMagnitudeAngle
  cfblk8 : Rounding
  cfblk9 : ComplexToRealImag
  cfblk2 : Outport
  wires:
  cfblk7/1 -> cfblk5/1
  cfblk3/1 -> cfblk9/1
  cfblk4/1 -> cfblk2/1
  cfblk10/1 -> cfblk7/1
  cfblk7/2 -> cfblk13/1
  cfblk12/1 -> cfblk4/1
  cfblk1/1 -> cfblk12/1
  cfblk9/1 -> cfblk10/1
  cfblk14/1 -> cfblk6/1
  cfblk11/1 -> cfblk8/1
  cfblk13/1 -> cfblk6/2
  cfblk6/1 -> cfblk11/1
  cfblk10/2 -> cfblk15/1
  cfblk15/1 -> cfblk3/1

== system sampleModel2072_pp_difftest/cfblk54/cfblk11 ==
  cfblk1 : Inport
  cfblk10 : Sum  Inputs=+-
  cfblk11 : DotProduct  InputSameDT=on  OutDataTypeStr=Inherit: Inherit via internal rule
  cfblk12 : Bias  Bias=[20999146.131458]
  cfblk13 : Sin  TimeSource=Use external signal  SampleTime=0
  cfblk14 : Delay  SampleTime=1
  cfblk15 : Delay  SampleTime=1
  cfblk3 : pid_lib/PID Controller (2DOF)  Controller=PID  Form=Parallel  TimeDomain=Discrete-time  UseExternalTs=off  SampleTime=1  IntegratorMethod=Forward Euler  FilterMethod=Forward Euler  ControllerParametersSource=internal  P=1  I=1  D=0  UseFilter=on  N=100  b=1  c=1  TunerSelectOption=Transfer Function Based (PID Tuner App)  InitialConditionSource=internal  InitialConditionForIntegrator=0  InitialConditionForFilter=0  DifferentiatorICPrevScaledInput=0  ExternalReset=none  TrackingMode=off  Kt=1  LimitOutput=off  SatLimitsSource=internal  UpperSaturationLimit=inf  LowerSaturationLimit=-inf  LinearizeAsGain=off  AntiWindupMode=none  Kb=1  POutMin=[]  POutMax=[]  IOutMin=[]  IOutMax=[]  DOutMin=[]  DOutMax=[]  NOutMin=[]  NOutMax=[]  bOutMin=[]  bOutMax=[]  cOutMin=[]  cOutMax=[]  SumOutMin=[]  SumOutMax=[]  SaturationOutMin=[]  SaturationOutMax=[]  PParamMin=[]  PParamMax=[]  IParamMin=[]  IParamMax=[]  DParamMin=[]  DParamMax=[]  NParamMin=[]  NParamMax=[]  bParamMin=[]  bParamMax=[]  cParamMin=[]  cParamMax=[]  KbParamMin=[]  KbParamMax=[]  KtParamMin=[]  KtParamMax=[]  KbOutMin=[]  KbOutMax=[]  KtOutMin=[]  KtOutMax=[]  IntegratorOutMin=[]  IntegratorOutMax=[]  FilterOutMin=[]  FilterOutMax=[]  SumI1OutMin=[]  SumI1OutMax=[]  SumI2OutMin=[]  SumI2OutMax=[]  SumI3OutMin=[]  SumI3OutMax=[]  SumI4OutMin=[]  SumI4OutMax=[]  SumDOutMin=[]  SumDOutMax=[]  Sum1OutMin=[]  Sum1OutMax=[]  Sum2OutMin=[]  Sum2OutMax=[]  Sum3OutMin=[]  Sum3OutMax=[]  DifferentiatorOutMin=[]  DifferentiatorOutMax=[]  FilterDiffOutCoefMin=[]  FilterDiffOutCoefMax=[]  ReciprocalOutMin=[]  ReciprocalOutMax=[]  SumDenOutMin=[]  SumDenOutMax=[]  SumNumOutMin=[]  SumNumOutMax=[]  DivideOutMin=[]  DivideOutMax=[]  UdiffTsProdOutMin=[]  UdiffTsProdOutMax=[]  NTsProdOutMin=[]  NTsProdOutMax=[]  UintegralTsProdOutMin=[]  UintegralTsProdOutMax=[]  UngainTsProdOutMin=[]  UngainTsProdOutMax=[]  IntegratorContinuousStateAttributes=''  IntegratorStateMustResolveToSignalObject=off  IntegratorRTWStateStorageClass=Auto  FilterContinuousStateAttributes=''  FilterStateMustResolveToSignalObject=off  FilterRTWStateStorageClass=Auto  ParallelPVariant=InternalParameters  IdealPVariant=Disabled  IVariant=InternalParameters  DVariant=InternalParameters  bVariant=InternalParameters  cVariant=InternalParameters  IntegratorVariant=Discrete  SatVariant=Disabled  AWVariant=Passthrough  PCopyVariant=Disabled  TRVariant=Disabled  FdbkBlocksVariant=Forward  IdealPFdbkVariant=Disabled  SatFdbkVariant=Disabled  DerivativeFilterVariant=ForwardEulerFilter  NVariant=InternalParameters  NCopyVariant=Disabled  FilterICVariant=InternalICsFilter  IntegratorICVariant=InternalICs  ExternalResetVariant=Disabled  TRSumVariant=Passthrough  SumFdbkVariant=Disabled  SumVariant=Sum_PID  TsampFilterVariant=InternalTs  TsampNgainVariant=Passthrough  TsampIntegralVariant=Passthrough  ExternalSaturationOutDataTypeStr=Inherit: Same as second input
      settings: SourceProductBaseCode=SL
  cfblk4 : simulink/Discrete/Transfer Fcn Lead or Lag  PoleZ=0.95  ZeroZ=0.75  ICPrevOutput=0.0  ICPrevInput=0.0  DoSatur=off
      settings: SourceProductBaseCode=SL
  cfblk5 : Sin  TimeSource=Use external signal  SampleTime=0
  cfblk6 : Sqrt  SaturateOnIntegerOverflow=on
  cfblk7 : Product
  cfblk8 : Gain  Gain=[125034912.605278]
  cfblk9 : simulink/Math Operations/MinMax Running Resettable  Function=min  vinit=0.0
  cfblk2 : Outport
  wires:
  cfblk6/1 -> cfblk9/1
  cfblk9/1 -> cfblk12/1, cfblk4/1
  cfblk12/1 -> cfblk11/1, cfblk5/1
  cfblk1/1 -> cfblk8/1, cfblk9/2
  cfblk4/1 -> cfblk13/1, cfblk11/2
  cfblk13/1 -> cfblk2/1
  cfblk7/1 -> cfblk6/1
  cfblk11/1 -> cfblk3/1
  cfblk8/1 -> cfblk10/1
  cfblk10/1 -> cfblk3/2, cfblk7/2
  cfblk3/1 -> cfblk14/1
  cfblk14/1 -> cfblk10/2
  cfblk5/1 -> cfblk15/1
  cfblk15/1 -> cfblk7/1

== system sampleModel2072_pp_difftest/cfblk54/cfblk12 ==
  cfblk1 : Inport
  cfblk10 : Bias  Bias=[-311026403.619236]
  cfblk11 : Abs
  cfblk12 : Delay  SampleTime=1
  cfblk13 : Delay  SampleTime=1
  cfblk3 : simulink/Discrete/Transfer Fcn Real Zero  ZeroZ=0.75  ICPrevInput=0.0  DoSatur=off
      settings: SourceProductBaseCode=SL
  cfblk4 : simulink/Discrete/Transfer Fcn Real Zero  ZeroZ=0.75  ICPrevInput=0.0  DoSatur=off
      settings: SourceProductBaseCode=SL
  cfblk5 : Gain  Gain=[330727659.340175]
  cfblk6 : Signum
  cfblk7 : Gain  Gain=[331123318.841085]
  cfblk8 : Squeeze
  cfblk9 : Abs
  cfblk2 : Outport
  wires:
  cfblk7/1 -> cfblk9/1
  cfblk9/1 -> cfblk5/1
  cfblk6/1 -> cfblk11/1
  cfblk1/1 -> cfblk2/1
  cfblk11/1 -> cfblk8/1
  cfblk8/1 -> cfblk7/1
  cfblk3/1 -> cfblk10/1
  cfblk4/1 -> cfblk6/1
  cfblk10/1 -> cfblk12/1
  cfblk12/1 -> cfblk3/1
  cfblk5/1 -> cfblk13/1
  cfblk13/1 -> cfblk4/1

== system sampleModel2072_pp_difftest/cfblk54/cfblk13 ==
  cfblk1 : Inport
  cfblk10 : simulink/Math Operations/MinMax Running Resettable  Function=min  vinit=0.0
  cfblk11 : Sum  Inputs=|++
  cfblk12 : Rounding
  cfblk13 : Sin  TimeSource=Use external signal  SampleTime=0
  cfblk14 : ComplexToRealImag
  cfblk15 : simulink/Math Operations/Slider Gain  gain=1  low=0  high=2
  cfblk16 : Sqrt  SaturateOnIntegerOverflow=on
  cfblk17 : Delay  SampleTime=1
  cfblk18 : Delay  SampleTime=1
  cfblk3 : Delay  DelayLengthSource=Input port  SampleTime=1
      settings: InputPortMap=u0,p1
  cfblk4 : simulink/Discrete/Transfer Fcn Lead or Lag  PoleZ=0.95  ZeroZ=0.75  ICPrevOutput=0.0  ICPrevInput=0.0  DoSatur=off
      settings: SourceProductBaseCode=SL
  cfblk5 : simulink/Discrete/Transfer Fcn First Order  PoleZ=0.95  ICPrevOutput=0.0  DoSatur=off
  cfblk6 : DiscreteZeroPole  Poles=[0 0.5]  Gain=1
  cfblk7 : simulink/Math Operations/Slider Gain  gain=1  low=0  high=2
  cfblk8 : PermuteDimensions
  cfblk9 : Product  Inputs=*
  cfblk2 : Outport
  wires:
  cfblk7/1 -> cfblk9/1, cfblk3/2
  cfblk4/1 -> cfblk10/1, cfblk13/1
  cfblk14/1 -> cfblk16/1
  cfblk11/1 -> cfblk3/1
  cfblk12/1 -> cfblk15/1
  cfblk5/1 -> cfblk2/1
  cfblk16/1 -> cfblk5/1
  cfblk10/1 -> cfblk7/1
  cfblk9/1 -> cfblk8/1
  cfblk8/1 -> cfblk12/1
  cfblk1/1 -> cfblk14/1
  cfblk14/2 -> cfblk10/2
  cfblk15/1 -> cfblk11/2
  cfblk3/1 -> cfblk6/1
  cfblk6/1 -> cfblk17/1
  cfblk17/1 -> cfblk11/1
  cfblk13/1 -> cfblk18/1
  cfblk18/1 -> cfblk4/1

== system sampleModel2072_pp_difftest/cfblk54/cfblk8 ==
  cfblk1 : Inport
  cfblk10 : Reshape
  cfblk11 : Sin  TimeSource=Use external signal  SampleTime=0
  cfblk12 : Sum  Inputs=|++
  cfblk13 : Rounding
  cfblk14 : simulink/Math Operations/MinMax Running Resettable  Function=min  vinit=0.0
  cfblk15 : Gain  Gain=[-489725140.841639]
  cfblk16 : Constant  Value=[-256347808.612234]  SampleTime=1
  cfblk17 : Delay  SampleTime=1
  cfblk3 : simulink/Discrete/Difference  ICPrevInput=0.0  OutMin=[]  OutMax=[]  OutDataTypeStr=Inherit: Inherit via back propagation  OutDataType=fixdt(1, 16)  OutScaling=2^-10  DoSatur=off
  cfblk4 : simulink/Discrete/Difference  ICPrevInput=0.0  OutMin=[]  OutMax=[]  OutDataTypeStr=Inherit: Inherit via back propagation  OutDataType=fixdt(1, 16)  OutScaling=2^-10  DoSatur=off
  cfblk5 : simulink/Discrete/Tapped Delay  vinit=0.0  samptime=-1  NumDelays=1  DelayOrder=Oldest  includeCurrent=off
  cfblk6 : simulink/Discrete/Transfer Fcn Lead or Lag  PoleZ=0.95  ZeroZ=0.75  ICPrevOutput=0.0  ICPrevInput=0.0  DoSatur=off
      settings: SourceProductBaseCode=SL
  cfblk7 : UnaryMinus
  cfblk8 : Math  Operator=magnitude^2  SaturateOnIntegerOverflow=on
  cfblk9 : Product  Inputs=**
  cfblk2 : Outport
  wires:
  cfblk11/1 -> cfblk7/1
  cfblk12/1 -> cfblk6/1
  cfblk7/1 -> cfblk8/1, cfblk15/1
  cfblk8/1 -> cfblk14/1
  cfblk14/1 -> cfblk2/1
  cfblk15/1 -> cfblk13/1
  cfblk16/1 -> cfblk11/1
  cfblk4/1 -> cfblk3/1
  cfblk1/1 -> cfblk12/1
  cfblk5/1 -> cfblk12/2, cfblk10/1
  cfblk9/1 -> cfblk4/1
  cfblk13/1 -> cfblk9/1
  cfblk6/1 -> cfblk9/2
  cfblk3/1 -> cfblk14/2
  cfblk10/1 -> cfblk17/1
  cfblk17/1 -> cfblk5/1

== system sampleModel2072_pp_difftest/cfblk54/cfblk9 ==
  cfblk1 : Inport
  cfblk10 : Signum
  cfblk11 : Sqrt  Operator=rSqrt  AlgorithmType=Newton-Raphson  SaturateOnIntegerOverflow=on
  cfblk12 : simulink/Math Operations/MinMax Running Resettable  Function=min  vinit=0.0
  cfblk13 : DotProduct  InputSameDT=on  OutDataTypeStr=Inherit: Inherit via internal rule
  cfblk14 : Constant  Value=[879636162.358787]  SampleTime=1
  cfblk15 : Delay  SampleTime=1
  cfblk16 : Delay  SampleTime=1
  cfblk3 : UnitDelay  HasFrameUpgradeWarning=on
  cfblk4 : simulink/Discrete/Transfer Fcn Lead or Lag  PoleZ=0.95  ZeroZ=0.75  ICPrevOutput=0.0  ICPrevInput=0.0  DoSatur=off
      settings: SourceProductBaseCode=SL
  cfblk5 : DiscreteZeroPole  Poles=[0 0.5]  Gain=1
  cfblk6 : Math  Operator=pow  SaturateOnIntegerOverflow=on
  cfblk7 : Sum  Inputs=+
  cfblk8 : simulink/Math Operations/Slider Gain  gain=1  low=0  high=2
  cfblk9 : simulink/Math Operations/MinMax Running Resettable  Function=min  vinit=0.0
  cfblk2 : Outport
  wires:
  cfblk6/1 -> cfblk5/1
  cfblk13/1 -> cfblk10/1
  cfblk10/1 -> cfblk12/1
  cfblk4/1 -> cfblk11/1, cfblk16/1
  cfblk3/1 -> cfblk9/1
  cfblk9/1 -> cfblk4/1
  cfblk1/1 -> cfblk13/1, cfblk6/2
  cfblk14/1 -> cfblk9/2
  cfblk8/1 -> cfblk13/2
  cfblk11/1 -> cfblk8/1
  cfblk7/1 -> cfblk2/1, cfblk6/1
  cfblk12/1 -> cfblk7/1
  cfblk5/1 -> cfblk15/1
  cfblk15/1 -> cfblk12/2
  cfblk16/1 -> cfblk3/1

== system sampleModel2072_pp_difftest/cfblk55/cfblk11 ==
  cfblk1 : Inport
  cfblk10 : Delay  SampleTime=1
  cfblk11 : Delay  SampleTime=1
  cfblk3 : simulink/Discrete/Tapped Delay  vinit=0.0  samptime=-1  NumDelays=1  DelayOrder=Oldest  includeCurrent=off
  cfblk4 : pid_lib/PID Controller (2DOF)  Controller=PID  Form=Parallel  TimeDomain=Discrete-time  UseExternalTs=off  SampleTime=1  IntegratorMethod=Forward Euler  FilterMethod=Forward Euler  ControllerParametersSource=internal  P=1  I=1  D=0  UseFilter=on  N=100  b=1  c=1  TunerSelectOption=Transfer Function Based (PID Tuner App)  InitialConditionSource=internal  InitialConditionForIntegrator=0  InitialConditionForFilter=0  DifferentiatorICPrevScaledInput=0  ExternalReset=none  TrackingMode=off  Kt=1  LimitOutput=off  SatLimitsSource=internal  UpperSaturationLimit=inf  LowerSaturationLimit=-inf  LinearizeAsGain=off  AntiWindupMode=none  Kb=1  POutMin=[]  POutMax=[]  IOutMin=[]  IOutMax=[]  DOutMin=[]  DOutMax=[]  NOutMin=[]  NOutMax=[]  bOutMin=[]  bOutMax=[]  cOutMin=[]  cOutMax=[]  SumOutMin=[]  SumOutMax=[]  SaturationOutMin=[]  SaturationOutMax=[]  PParamMin=[]  PParamMax=[]  IParamMin=[]  IParamMax=[]  DParamMin=[]  DParamMax=[]  NParamMin=[]  NParamMax=[]  bParamMin=[]  bParamMax=[]  cParamMin=[]  cParamMax=[]  KbParamMin=[]  KbParamMax=[]  KtParamMin=[]  KtParamMax=[]  KbOutMin=[]  KbOutMax=[]  KtOutMin=[]  KtOutMax=[]  IntegratorOutMin=[]  IntegratorOutMax=[]  FilterOutMin=[]  FilterOutMax=[]  SumI1OutMin=[]  SumI1OutMax=[]  SumI2OutMin=[]  SumI2OutMax=[]  SumI3OutMin=[]  SumI3OutMax=[]  SumI4OutMin=[]  SumI4OutMax=[]  SumDOutMin=[]  SumDOutMax=[]  Sum1OutMin=[]  Sum1OutMax=[]  Sum2OutMin=[]  Sum2OutMax=[]  Sum3OutMin=[]  Sum3OutMax=[]  DifferentiatorOutMin=[]  DifferentiatorOutMax=[]  FilterDiffOutCoefMin=[]  FilterDiffOutCoefMax=[]  ReciprocalOutMin=[]  ReciprocalOutMax=[]  SumDenOutMin=[]  SumDenOutMax=[]  SumNumOutMin=[]  SumNumOutMax=[]  DivideOutMin=[]  DivideOutMax=[]  UdiffTsProdOutMin=[]  UdiffTsProdOutMax=[]  NTsProdOutMin=[]  NTsProdOutMax=[]  UintegralTsProdOutMin=[]  UintegralTsProdOutMax=[]  UngainTsProdOutMin=[]  UngainTsProdOutMax=[]  IntegratorContinuousStateAttributes=''  IntegratorStateMustResolveToSignalObject=off  IntegratorRTWStateStorageClass=Auto  FilterContinuousStateAttributes=''  FilterStateMustResolveToSignalObject=off  FilterRTWStateStorageClass=Auto  ParallelPVariant=InternalParameters  IdealPVariant=Disabled  IVariant=InternalParameters  DVariant=InternalParameters  bVariant=InternalParameters  cVariant=InternalParameters  IntegratorVariant=Discrete  SatVariant=Disabled  AWVariant=Passthrough  PCopyVariant=Disabled  TRVariant=Disabled  FdbkBlocksVariant=Forward  IdealPFdbkVariant=Disabled  SatFdbkVariant=Disabled  DerivativeFilterVariant=ForwardEulerFilter  NVariant=InternalParameters  NCopyVariant=Disabled  FilterICVariant=InternalICsFilter  IntegratorICVariant=InternalICs  ExternalResetVariant=Disabled  TRSumVariant=Passthrough  SumFdbkVariant=Disabled  SumVariant=Sum_PID  TsampFilterVariant=InternalTs  TsampNgainVariant=Passthrough  TsampIntegralVariant=Passthrough  ExternalSaturationOutDataTypeStr=Inherit: Same as second input
      settings: SourceProductBaseCode=SL
  cfblk5 : DiscreteTransferFcn  SampleTime=1
  cfblk6 : simulink/Math Operations/MinMax Running Resettable  Function=min  vinit=0.0
  cfblk7 : ComplexToMagnitudeAngle
  cfblk8 : Reshape
  cfblk9 : Polyval  Coefs=[ +2.081618890e-019, -1.441693666e-014, +4.719686976e-010, -8.536869453e-006, +1.621573104e-001, -8.087801117e+001 ]
  cfblk2 : Outport
  wires:
  cfblk4/1 -> cfblk3/1
  cfblk7/1 -> cfblk2/1
  cfblk6/1 -> cfblk8/1
  cfblk5/1 -> cfblk9/1, cfblk4/2
  cfblk1/1 -> cfblk6/1
  cfblk9/1 -> cfblk7/1
  cfblk8/1 -> cfblk4/1
  cfblk3/1 -> cfblk10/1
  cfblk10/1 -> cfblk6/2
  cfblk7/2 -> cfblk11/1
  cfblk11/1 -> cfblk5/1

== system sampleModel2072_pp_difftest/cfblk55/cfblk12 ==
  cfblk1 : Inport
  cfblk10 : DotProduct  InputSameDT=on  OutDataTypeStr=Inherit: Inherit via internal rule
  cfblk11 : Trigonometry
  cfblk12 : Sum  Inputs=|++
  cfblk13 : Abs
  cfblk14 : Sqrt  SaturateOnIntegerOverflow=on
  cfblk15 : PermuteDimensions
  cfblk16 : Constant  Value=[-683900231.411340]  SampleTime=1
  cfblk17 : Delay  SampleTime=1
  cfblk18 : Delay  SampleTime=1
  cfblk3 : DiscreteFilter  SampleTime=1
  cfblk4 : DiscreteFir  SampleTime=1
  cfblk5 : DiscreteFir  SampleTime=1
  cfblk6 : DiscreteFir  SampleTime=1
  cfblk7 : Sin  TimeSource=Use external signal  SampleTime=0
  cfblk8 : UnaryMinus
  cfblk9 : Assignment  DiagnosticForDimensions=Warning  IndexOptions=Index vector (dialog)  Indices=1  OutputSizes=1
  cfblk2 : Outport
  wires:
  cfblk5/1 -> cfblk8/1
  cfblk12/1 -> cfblk14/1
  cfblk6/1 -> cfblk12/1
  cfblk1/1 -> cfblk6/1
  cfblk16/1 -> cfblk2/1, cfblk10/2
  cfblk9/1 -> cfblk13/1
  cfblk3/1 -> cfblk10/1, cfblk4/1
  cfblk13/1 -> cfblk5/1
  cfblk8/1 -> cfblk7/1
  cfblk15/1 -> cfblk11/1
  cfblk7/1 -> cfblk15/1
  cfblk4/1 -> cfblk9/2
  cfblk14/1 -> cfblk3/1
  cfblk10/1 -> cfblk17/1
  cfblk17/1 -> cfblk12/2
  cfblk11/1 -> cfblk18/1
  cfblk18/1 -> cfblk9/1

== system sampleModel2072_pp_difftest/cfblk56/cfblk13 ==
  cfblk1 : Inport
  cfblk3 : DiscreteIntegrator  ICPrevOutput=DiscIntNeverNeededParam  ICPrevScaledInput=DiscIntNeverNeededParam
  cfblk4 : Delay  DelayLengthSource=Input port  SampleTime=1
      settings: InputPortMap=u0,p1
  cfblk5 : Math  Operator=magnitude^2  SaturateOnIntegerOverflow=on
  cfblk6 : Sum  Inputs=+
  cfblk7 : Gain  Gain=[-939956077.062767]
  cfblk8 : Product  Inputs=**
  cfblk9 : Delay  SampleTime=1
  cfblk2 : Outport
  wires:
  cfblk4/1 -> cfblk2/1
  cfblk1/1 -> cfblk8/1
  cfblk5/1 -> cfblk3/1
  cfblk7/1 -> cfblk5/1
  cfblk8/1 -> cfblk7/1, cfblk6/1
  cfblk6/1 -> cfblk4/2, cfblk9/1
  cfblk3/1 -> cfblk4/1
  cfblk9/1 -> cfblk8/2

== system sampleModel2072_pp_difftest/cfblk56/cfblk14 ==
  cfblk1 : Inport
  cfblk10 : Sqrt  SaturateOnIntegerOverflow=on
  cfblk11 : PermuteDimensions
  cfblk12 : Product  Inputs=*
  cfblk13 : Sqrt  Operator=rSqrt  AlgorithmType=Newton-Raphson  SaturateOnIntegerOverflow=on
  cfblk14 : Trigonometry
  cfblk15 : Delay  SampleTime=1
  cfblk16 : Delay  SampleTime=1
  cfblk3 : DiscreteTransferFcn  SampleTime=1
  cfblk4 : DiscreteFilter  SampleTime=1
  cfblk5 : DiscreteIntegrator  ICPrevOutput=DiscIntNeverNeededParam  ICPrevScaledInput=DiscIntNeverNeededParam
  cfblk6 : Delay  DelayLengthSource=Input port  SampleTime=1
      settings: InputPortMap=u0,p1
  cfblk7 : UnitDelay  HasFrameUpgradeWarning=on
  cfblk8 : Sum
  cfblk9 : ComplexToMagnitudeAngle
  cfblk2 : Outport
  wires:
  cfblk9/1 -> cfblk2/1
  cfblk13/1 -> cfblk5/1
  cfblk9/2 -> cfblk13/1
  cfblk14/1 -> cfblk9/1
  cfblk7/1 -> cfblk3/1
  cfblk6/1 -> cfblk10/1
  cfblk12/1 -> cfblk4/1, cfblk14/1
  cfblk3/1 -> cfblk11/1
  cfblk11/1 -> cfblk8/2
  cfblk8/1 -> cfblk12/1
  cfblk1/1 -> cfblk7/1
  cfblk4/1 -> cfblk6/2
  cfblk10/1 -> cfblk15/1
  cfblk15/1 -> cfblk6/1
  cfblk5/1 -> cfblk16/1
  cfblk16/1 -> cfblk8/1
